simulink model "FFM_Punch"  (R2017a)
settings: Solver=ode3  StartTime=0.0  StopTime=timesteps  FixedStep=data.SIM.Ts  RelTol=1e-3  EnableMultiTasking=on
values from neighbouring files (symbols this model uses):
  data =     [dakota_config.mat]
  downshift_map = data.TCU.upshift.veh_spd_default    [Simulation_results.m]
  upshift_map = data.TCU.upshift.veh_spd_default    [Simulation_results.m]
undefined symbols (not defined in the file or in its folder): air_density, Cd, DiscIntNeverNeededParam, fr_crankshaft, fr_speed_values, g, i_FD, ICE, Low_Ratio, M_Eng_Max, M_Eng_Max_Max, M_Eng_Max_Rpm, mt2m_f, mu_Roll_C0, mu_Roll_C1, mu_Roll_C2, Mv, n_Idle_Eng, Overdrive_Ratio, Re, S_eff_drag, Ts
(part 10 of 15)

== system FFM_Punch/Driver Interface/Driver Model/Driver Pedals Determination/Brake_Pedal_Determination ==
  M_Driv : Inport
  M_eng_drvSat : Inport  Port=2
  r_Overall : Inport  Port=3
  b_neut : Inport  Port=4
  Constant : Constant  Tag=Controls_Lib  Description=constant  Value=Value  OutMin=OutMin  OutMax=OutMax  OutDataTypeStr=single  SampleTime=SampleTime  FramePeriod=FramePeriod  mask(Constant){Value=0, VectorParams1D=on, SampleTime=-1, FramePeriod=inf, OutMin=[], OutMax=[], OutDataTypeStr=single, LockScale=off}
      mask prompts: Value "Simulink:blkprm_prompts:ConstConstValue"; VectorParams1D "Simulink:blkprm_prompts:AllSrcsVector1D"; SampleTime "Simulink:blkprm_prompts:AllSrcBlksSampleTime"; FramePeriod "Simulink:blkprm_prompts:AllSrcBlksFramePeriod"; OutMin "Simulink:blkprm_prompts:OutputDesignMin"; OutMax "Simulink:blkprm_prompts:OutputDesignMax"; OutDataTypeStr "Simulink:blkprm_prompts:OUTPUT_UNIFIEDDATATYPE"; LockScale "Simulink:blkprm_prompts:LockScale"
      mask help: Output the constant specified by the 'Constant value' parameter.
      mask Help: web([fileparts(which('Lib_built')) filesep 'hlp' filesep 'lib_constant' '.html'], '-helpbrowser')
      mask TypeOptions Value: Value
      mask TypeOptions VectorParams1D: VectorParams1D
      mask TypeOptions SampleTime: SampleTime
      mask TypeOptions FramePeriod: FramePeriod
      mask TypeOptions OutMin: OutMin
      mask TypeOptions OutMax: OutMax
      mask TypeOptions OutDataTypeStr: OutDataTypeStr
      mask TypeOptions LockScale: LockScale
      mask DialogControl ParameterTabVar0 Prompt: Main
      mask Display: disp(get_param(gcb,'Value'))
  Constant2 : Constant  Value=0  OutDataTypeStr=single
  Constant3 : Constant  Value=-10000  OutDataTypeStr=single
  Gain3 : Gain  Gain=-1
  Product1 : Product  Inputs=**  RndMeth=Zero
  Saturation Dynamic : Subsystem  mask(Saturation Dynamic){OutMin=[], OutMax=[], OutDataTypeStr=single, OutputDataTypeScalingMode=single, OutDataType=sfix(16), OutScaling=2^-10, LockScale=off, RndMeth=Floor, DoSatur=off}
      mask prompts: OutMin "Simulink:masks:OutputMinimum_MP"; OutMax "Simulink:masks:OutputMaximum_MP"; OutDataTypeStr "Simulink:masks:OutputDataType_MP"; OutputDataTypeScalingMode "Simulink:masks:OutputDataTypeMode_MP"; OutDataType "Simulink:masks:OutputDataTypeegFixdt116Fixdtsingle_MP"; OutScaling "Simulink:masks:OutputScalingSlopeEg29OrSlopeBias_MP"; LockScale "Simulink:masks:LockOutputDataTypeAgainstFxpTools_MP"; RndMeth "Simulink:masks:IntegerRoundingMode_MP"; DoSatur "Simulink:masks:SaturateOnIntegerOverflow_MP"
      mask help: Simulink:masks:SaturationDynamic_MD
      mask init: same as FFM_Punch/Driver Interface/Driver Model-_old/Driver Pedal Behaviour/Saturation Dynamic
      mask Callback OutDataTypeStr: fixptdialog(gcbh)
      mask TypeOptions OutputDataTypeScalingMode: double | single | int8 | uint8 | int16 | uint16 | int32 | uint32 | Specify via dialog | Same as second input
      mask Callback OutputDataTypeScalingMode: fixptdialog(gcbh)
      mask Callback OutDataType: fixptdialog(gcbh)
      mask TypeOptions RndMeth: Simulink:masks:Ceiling | Simulink:masks:Convergent | Simulink:masks:Floor | Simulink:masks:Nearest | Simulink:masks:Round | Simulink:masks:Simplest | Simulink:masks:Zero
      mask Display: plot([0.15 0.85],[.5 .5],[.5 .5],[0.05 0.95],0.15+0.7*[0 .25 .75 1],0.05+0.9*[.25 .25 .75 .75]);
  Sum2 : Sum  Inputs=-+  OutDataTypeStr=Inherit: Inherit via back propagation
  Switch : Switch  Tag=Controls_Lib  Description=Switch  Criteria=u2 ~= 0  Threshold=Threshold  OutMin=OutMin  OutMax=OutMax  OutDataTypeStr=Inherit: Inherit via back propagation  RndMeth=Zero  ZeroCross=off  SampleTime=SampleTime  InputSameDT=on  mask(Switch){Criteria=u2 ~= 0, Threshold=0.5, ZeroCross=off, SampleTime=-1, InputSameDT=on, OutMin=[], OutMax=[], OutDataTypeStr=Inherit: Inherit via back propagation, LockScale=off, RndMeth=Zero, SaturateOnIntegerOverflow=off, AllowDiffInputSizes=off}
      mask prompts: Criteria "Criteria for passing first input:"; ZeroCross "Enable zero-crossing detection"; SampleTime "Sample time (-1 for inherited):"; InputSameDT "Require all data port inputs to have the same data type"; OutMin "Output minimum:"; OutMax "Output maximum:"; OutDataTypeStr "Output data type:"; LockScale "Lock output data type setting against changes by the fixed-point tools"; RndMeth "Integer rounding mode:"; SaturateOnIntegerOverflow "Saturate on integer overflow"; AllowDiffInputSizes "Allow different data input sizes (Results in variable-size output signal)"
      mask help:
      | Pass through input 1 when input 2 is not equal to 0. Otherwise, pass through input 3.  The inputs are numbered top to bottom (or left to right). The input 1 pass-through criteria are input 2 not equal to 0;
      | The first and third input ports are data ports, and the second input port is the control port. The control port signal should always be a boolean signal.
      mask Help: web([fileparts(which('Lib_built')) filesep 'hlp' filesep 'lib_Switch' '.html'], '-helpbrowser')
      mask TypeOptions Criteria: Criteria
      mask TypeOptions Threshold: Threshold
      mask TypeOptions ZeroCross: ZeroCross
      mask TypeOptions SampleTime: SampleTime
      mask TypeOptions InputSameDT: InputSameDT
      mask TypeOptions OutMin: OutMin
      mask TypeOptions OutMax: OutMax
      mask TypeOptions OutDataTypeStr: OutDataTypeStr
      mask TypeOptions LockScale: LockScale
      mask TypeOptions RndMeth: RndMeth
      mask TypeOptions SaturateOnIntegerOverflow: SaturateOnIntegerOverflow
      mask TypeOptions AllowDiffInputSizes: AllowDiffInputSizes
  "brake request -> brake pedal" : Lookup  InputValues=|  Table=|  LookUpMeth=Interpolation-Use End Values
      InputValues=|
      | [0
      | 
      | 
      | 200
      | 
      | 
      | 400
      | 
      | 
      | 600
      | 
      | 
      | 800
      | 
      | 
      | 1000
      | 
      | 
      | 1200
      | 
      | 
      | 1400
      | 
      | 1600
      | 
      | 
      | 1800
      | 
      | 2000]*2
      Table=|
      | [0
      | 
      | 
      | 10
      | 
      | 
      | 20
      | 
      | 
      | 30
      | 
      | 
      | 40
      | 
      | 
      | 50
      | 
      | 
      | 60
      | 
      | 
      | 70
      | 
      | 
      | 80
      | 
      | 
      | 90
      | 
      | 
      | 100]
  Driver_Brake_Request_Dcy : Outport
  wires:
  r_Overall/1 -> [r_Overall]
  M_eng_drvSat/1 -> [M_eng_drvSat]
  M_Driv/1 -> [M_Driv]
  [Driver_Brake_Request_Dcy] -> Driver_Brake_Request_Dcy/1
  Saturation Dynamic/1(y) -> Gain3/1
  Constant2/1 -> Saturation Dynamic/1(up)
  Constant3/1 -> Saturation Dynamic/3(lo)
  [M_Driv] -> Sum2/2  "wheel"
  Sum2/1 -> Saturation Dynamic/2(u)
  Gain3/1 -> "brake request -> brake pedal"/1
  "brake request -> brake pedal"/1 -> [Driver_Brake_Request_Dcy]
  [r_Overall] -> Product1/1
  [M_eng_drvSat] -> Product1/2
  Constant/1 -> Switch/3
  b_neut/1 -> Switch/2
  Switch/1 -> Sum2/1
  Product1/1 -> Switch/1

== system FFM_Punch/Driver Interface/Driver Model/Driver Pedals Determination/Preliminary_Calculations ==
  M_Driv : Inport
  n_Eng : Inport  Port=2
  r_Overall : Inport  Port=3
  v_Veh : Inport  Port=4
  Constant1 : Constant  Value=10000  OutDataTypeStr=Inherit: Inherit via back propagation
  Constant16 : Constant  Value=-100000  OutDataTypeStr=Inherit: Inherit via back propagation
  Product : Product  Inputs=*/  RndMeth=Zero
  RateLimiter : Subsystem  Tag=Controls_Lib  Description=RateLimiter  mask(Rate Limiter Dynamic){}
      mask help:
      | Limit upper and lower rates of the input signal based on the UL and LL. The rate is not limited at the first instance, output is same as the input at the first instance. 'Issat' is set to TRUE if the rate of the input signal is saturated.
      |
      | Note: The upper limit should be at least greater than or equal to the lower limit to guarantee the intended functionality.
      |
      | Inputs:
      | UL- Single [Inp/Ts]
      | Inp- Single [-]
      | LL- Single [Inp/Ts]
      |
      | outputs:
      | Out-Single [-]
      | Issat-Boolean [-]
      |
      | Where, Ts is the sample time of the model
      mask Help: web([fileparts(which('Lib_discontious')) filesep 'hlp' filesep 'lib_RateLim.html'], '-helpbrowser')
      mask Display: plot([0.15 0.95],[.5 .5],[.5 .5],[0.05 0.95],0.05+0.9*[.2 .8],0.05+0.9*[0 1]);
  Saturation1 : Saturate  UpperLimit=50  LowerLimit=data.SIM.eps
  Terminator1 : Terminator
      settings: Tag=Controls_Lib  Description=Terminator
  Terminator2 : Terminator
      settings: Tag=Controls_Lib  Description=Terminator
  Terminator3 : Terminator
      settings: Tag=Controls_Lib  Description=Terminator
  M_eng_drvSat : Outport
  wires:
  r_Overall/1 -> [r_Overall]
  n_Eng/1 -> Terminator1/1
  M_Driv/1 -> [M_Driv]
  [M_eng_drvSat] -> M_eng_drvSat/1
  Product/1 -> RateLimiter/2(Inp)  "engine"
  [M_Driv] -> Product/1
  Saturation1/1 -> Product/2
  [r_Overall] -> Saturation1/1
  Constant16/1 -> RateLimiter/3(LL)
  RateLimiter/1(Out) -> [M_eng_drvSat]
  v_Veh/1 -> Terminator2/1
  Constant1/1 -> RateLimiter/1(UL)
  RateLimiter/2(Issat) -> Terminator3/1

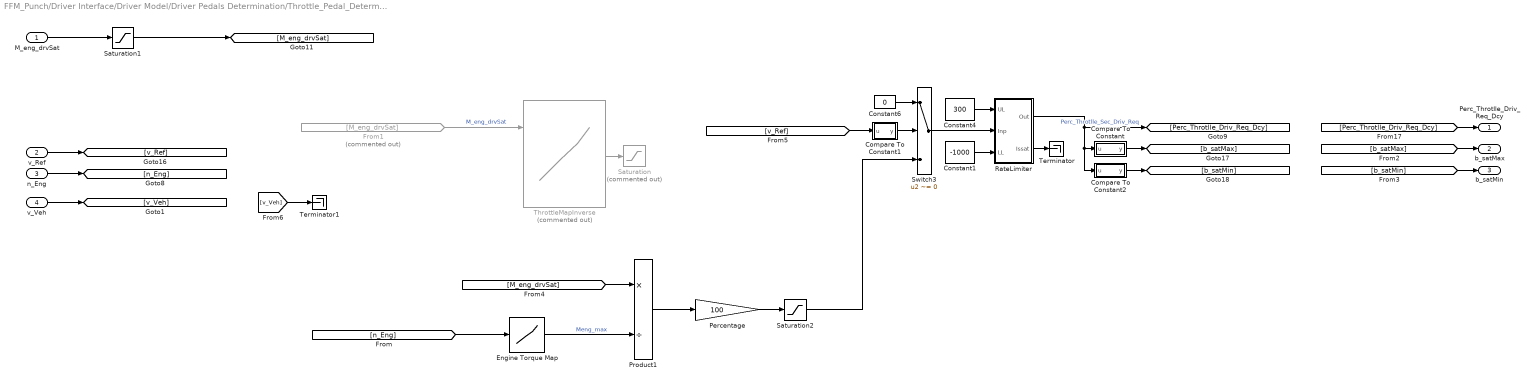
== system FFM_Punch/Driver Interface/Driver Model/Driver Pedals Determination/Throttle_Pedal_Determination ==
  M_eng_drvSat : Inport
  v_Ref : Inport  Port=2
  n_Eng : Inport  Port=3
  v_Veh : Inport  Port=4
  Compare To Constant : Subsystem  mask(Compare To Constant){relop=>=, const=100, OutDataTypeStr=boolean, ZeroCross=on}
      mask prompts: relop "Simulink:masks:Operator_MP"; const "Simulink:masks:ConstantValue_MP"; OutDataTypeStr "Simulink:masks:OutputDataType_MP"; ZeroCross "Simulink:masks:EnableZerocrossingDetection_MP"
      mask help: Simulink:masks:CompareToConstant_MD
      mask init: same as FFM_Punch/Driver Interface/Compare To Constant3
      mask TypeOptions relop: == | ~= | < | <= | >= | >
      mask TypeOptions OutDataTypeStr: Simulink:masks:uint8 | Simulink:masks:boolean
      mask Callback ZeroCross: sl('zeroCrossEnable', gcbh);
      mask Display: disp(str)
  Compare To Constant1 : Subsystem  mask(Compare To Constant){relop=<, const=1, OutDataTypeStr=boolean, ZeroCross=off}
      mask prompts: relop "Simulink:masks:Operator_MP"; const "Simulink:masks:ConstantValue_MP"; OutDataTypeStr "Simulink:masks:OutputDataType_MP"; ZeroCross "Simulink:masks:EnableZerocrossingDetection_MP"
      mask help: Simulink:masks:CompareToConstant_MD
      mask init: same as FFM_Punch/Driver Interface/Compare To Constant3
      mask TypeOptions relop: == | ~= | < | <= | >= | >
      mask TypeOptions OutDataTypeStr: Simulink:masks:uint8 | Simulink:masks:boolean
      mask Callback ZeroCross: sl('zeroCrossEnable', gcbh);
      mask Display: disp(str)
  Compare To Constant2 : Subsystem  mask(Compare To Constant){relop=<=, const=0, OutDataTypeStr=boolean, ZeroCross=on}
      mask prompts: relop "Simulink:masks:Operator_MP"; const "Simulink:masks:ConstantValue_MP"; OutDataTypeStr "Simulink:masks:OutputDataType_MP"; ZeroCross "Simulink:masks:EnableZerocrossingDetection_MP"
      mask help: Simulink:masks:CompareToConstant_MD
      mask init: same as FFM_Punch/Driver Interface/Compare To Constant3
      mask TypeOptions relop: == | ~= | < | <= | >= | >
      mask TypeOptions OutDataTypeStr: Simulink:masks:uint8 | Simulink:masks:boolean
      mask Callback ZeroCross: sl('zeroCrossEnable', gcbh);
      mask Display: disp(str)
  Constant1 : Constant  Value=-1000  OutDataTypeStr=single
  Constant4 : Constant  Value=300  OutDataTypeStr=single
  Constant6 : Constant  Value=0  OutDataTypeStr=Inherit: Inherit via back propagation
  Engine Torque Map : Lookup  InputValues=ICE.M_iceMax_XA.Value  Table=ICE.M_iceMax_M1.Value  LookUpMeth=Interpolation-Use End Values
  From1 : From  Commented=on  GotoTag=M_eng_drvSat
  Percentage : Gain  Gain=100
  Product1 : Product  Inputs=*/  SaturateOnIntegerOverflow=on  RndMeth=Zero  InputSameDT=on  OutDataTypeStr=Inherit: Same as first input
  RateLimiter : Subsystem  Tag=Controls_Lib  Description=RateLimiter  mask(Rate Limiter Dynamic){}
      mask help:
      | Limit upper and lower rates of the input signal based on the UL and LL. The rate is not limited at the first instance, output is same as the input at the first instance. 'Issat' is set to TRUE if the rate of the input signal is saturated.
      |
      | Note: The upper limit should be at least greater than or equal to the lower limit to guarantee the intended functionality.
      |
      | Inputs:
      | UL- Single [Inp/Ts]
      | Inp- Single [-]
      | LL- Single [Inp/Ts]
      |
      | outputs:
      | Out-Single [-]
      | Issat-Boolean [-]
      |
      | Where, Ts is the sample time of the model
      settings: PreCopyFcn=error('This MBD-Library block is outdated and replaced with an updated version. Please use the updated block from the MBD-Library (outdated blocks are colored in red).')
      mask Help: web([fileparts(which('Lib_discontious')) filesep 'hlp' filesep 'lib_RateLim.html'], '-helpbrowser')
      mask Display: plot([0.15 0.95],[.5 .5],[.5 .5],[0.05 0.95],0.05+0.9*[.2 .8],0.05+0.9*[0 1]);
  Saturation : Saturate  Commented=on  UpperLimit=100  LowerLimit=0
  Saturation1 : Saturate  UpperLimit=max(ICE.M_iceMax_M1.Value)  LowerLimit=0
  Saturation2 : Saturate  UpperLimit=100  LowerLimit=0
  Switch3 : Switch  Criteria=u2 ~= 0  Threshold=0.5  RndMeth=Zero  InputSameDT=on
  Terminator : Terminator
      settings: Tag=Controls_Lib  Description=Terminator
  Terminator1 : Terminator
      settings: Tag=Controls_Lib  Description=Terminator
  ThrottleMapInverse : Lookup_n-D  Commented=on  BreakpointsForDimension1=PedalMapInv_Data(1,2:end)  BreakpointsForDimension2=PedalMapInv_Data(2:end,1)  IndexSearchMethod=Linear search  BeginIndexSearchUsingPreviousIndexResult=on  Table=PedalMapInv_Data(2:end,2:end)  UseLastTableValue=on  RndMeth=Simplest  InputSameDT=on
  Perc_Throtlle_Driv_Req_Dcy : Outport
  b_satMax : Outport  Port=2
  b_satMin : Outport  Port=3
  wires:
  v_Ref/1 -> [v_Ref]
  M_eng_drvSat/1 -> Saturation1/1
  [Perc_Throtlle_Driv_Req_Dcy] -> Perc_Throtlle_Driv_Req_Dcy/1
  From1/1 -> ThrottleMapInverse/1  "M_eng_drvSat"
  ThrottleMapInverse/1 -> Saturation/1
  Compare To Constant1/1(y) -> Switch3/2
  [v_Ref] -> Compare To Constant1/1(u)
  Constant6/1 -> Switch3/1
  Switch3/1 -> RateLimiter/2(Inp)
  Constant4/1 -> RateLimiter/1(UL)
  Constant1/1 -> RateLimiter/3(LL)
  RateLimiter/1(Out) -> [Perc_Throtlle_Driv_Req_Dcy], Compare To Constant/1(u), Compare To Constant2/1(u)  "Perc_Throtlle_Sec_Driv_Req"
  Compare To Constant/1(y) -> [b_satMax]
  Compare To Constant2/1(y) -> [b_satMin]
  [b_satMax] -> b_satMax/1
  [b_satMin] -> b_satMin/1
  n_Eng/1 -> [n_Eng]
  RateLimiter/2(Issat) -> Terminator/1
  v_Veh/1 -> [v_Veh]
  Saturation1/1 -> [M_eng_drvSat]
  [n_Eng] -> Engine Torque Map/1
  Engine Torque Map/1 -> Product1/2  "Meng_max"
  Product1/1 -> Percentage/1
  [M_eng_drvSat] -> Product1/1
  Percentage/1 -> Saturation2/1
  Saturation2/1 -> Switch3/3
  [v_Veh] -> Terminator1/1

== system FFM_Punch/Driver Interface/Driver Model/Final PID Computation/Anti windup ==
  b_satMax : Inport
  b_satMin : Inport  Port=2
  v_ErrorIn : Inport  Port=3
  Constant1 : Constant  Value=0  OutDataTypeStr=Inherit: Inherit via back propagation  SampleTime=-1
  Constant81 : Constant  Value=0  OutDataTypeStr=Inherit: Inherit via back propagation  SampleTime=-1
  MinMax1 : MinMax  Function=max  Inputs=2  OutDataTypeStr=Inherit: Inherit via back propagation
  MinMax8 : MinMax  Inputs=2  OutDataTypeStr=Inherit: Inherit via back propagation
  Switch : Switch  Threshold=1  OutDataTypeStr=Inherit: Inherit via back propagation
  Switch1 : Switch  Threshold=1  OutDataTypeStr=Inherit: Inherit via back propagation
  v_ErrorOut : Outport
  wires:
  v_ErrorIn/1 -> Switch/3, MinMax8/1
  b_satMax/1 -> Switch/2
  b_satMin/1 -> Switch1/2
  MinMax1/1 -> Switch1/1
  Switch/1 -> Switch1/3, MinMax1/1
  Constant1/1 -> MinMax1/2
  MinMax8/1 -> Switch/1
  Switch1/1 -> v_ErrorOut/1
  Constant81/1 -> MinMax8/2

== system FFM_Punch/Driver Interface/Driver Model/Final PID Computation/Compare To Constant3 ==
  u : Inport
  Compare : RelationalOperator  OutDataTypeStr=boolean  ZeroCross=off  RndMeth=Nearest  InputSameDT=on
  Constant : Constant  DisableCoverage=on  Value=const  OutDataTypeStr=Inherit: Inherit via back propagation
  y : Outport
  wires:
  u/1 -> Compare/1
  Constant/1 -> Compare/2
  Compare/1 -> y/1

== system FFM_Punch/Driver Interface/Driver Model/Final Pedal Coordination/RateLimiter ==
  UL : Inport  Tag=Controls_Lib_V1.0  OutDataTypeStr=single  Interpolate=off
  Inp : Inport  Tag=Controls_Lib_V1.0  Port=2  OutDataTypeStr=single  Interpolate=off
  LL : Inport  Tag=Controls_Lib_V1.0  Port=3  OutDataTypeStr=single  Interpolate=off
  AddSub : Sum  Tag=Controls_Lib_V1.0  Inputs=+-  CollapseDim=CollapseDim  AccumDataTypeStr=single  OutMin=OutMin  OutMax=OutMax  OutDataTypeStr=single  RndMeth=Nearest  SampleTime=SampleTime  InputSameDT=on  mask(AddSub){IconShape=rectangular, Inputs=+-, CollapseMode=All dimensions, CollapseDim=1, SampleTime=-1, InputSameDT=on, AccumDataTypeStr=single, OutMin=[], OutMax=[], OutDataTypeStr=single, LockScale=off, RndMeth=Nearest, SaturateOnIntegerOverflow=off}
      mask prompts: IconShape "Icon shape:"; Inputs "List of signs:"; CollapseMode "Sum over:"; CollapseDim "Dimension:"; SampleTime "Sample time (-1 for inherited):"; InputSameDT "Require all inputs to have the same data type"; AccumDataTypeStr "Accumulator data type:"; OutMin "Output minimum:"; OutMax "Output maximum:"; OutDataTypeStr "Output data type:"; LockScale "Lock data type settings against changes by the fixed-point tools"; RndMeth "Integer rounding mode:"; SaturateOnIntegerOverflow "Saturate on integer overflow"
      mask help:
      | Add or subtract inputs.  Specify one of the following:
      | a) string containing + or - for each input port, | for spacer between ports (e.g. ++|-|++)
      | b) scalar, >= 1, specifies the number of input ports to be summed.
      | When there is only one input port, add or subtract elements over all dimensions or one specified dimension
      mask Help: web([fileparts(which('Lib_built')) filesep 'hlp' filesep 'lib_AddSub' '.html'], '-helpbrowser')
      mask TypeOptions IconShape: IconShape
      mask TypeOptions Inputs: Inputs
      mask TypeOptions CollapseMode: CollapseMode
      mask TypeOptions CollapseDim: CollapseDim
      mask TypeOptions SampleTime: SampleTime
      mask TypeOptions InputSameDT: InputSameDT
      mask TypeOptions AccumDataTypeStr: AccumDataTypeStr
      mask TypeOptions OutMin: OutMin
      mask TypeOptions OutMax: OutMax
      mask TypeOptions OutDataTypeStr: OutDataTypeStr
      mask TypeOptions LockScale: LockScale
      mask TypeOptions RndMeth: RndMeth
      mask TypeOptions SaturateOnIntegerOverflow: SaturateOnIntegerOverflow
  AddSub1 : Sum  Tag=Controls_Lib_V1.0  CollapseDim=CollapseDim  AccumDataTypeStr=single  OutMin=OutMin  OutMax=OutMax  OutDataTypeStr=single  RndMeth=Nearest  SampleTime=SampleTime  InputSameDT=on  mask(AddSub){IconShape=rectangular, Inputs=++, CollapseMode=All dimensions, CollapseDim=1, SampleTime=-1, InputSameDT=on, AccumDataTypeStr=single, OutMin=[], OutMax=[], OutDataTypeStr=single, LockScale=off, RndMeth=Nearest, SaturateOnIntegerOverflow=off}
      mask prompts: IconShape "Icon shape:"; Inputs "List of signs:"; CollapseMode "Sum over:"; CollapseDim "Dimension:"; SampleTime "Sample time (-1 for inherited):"; InputSameDT "Require all inputs to have the same data type"; AccumDataTypeStr "Accumulator data type:"; OutMin "Output minimum:"; OutMax "Output maximum:"; OutDataTypeStr "Output data type:"; LockScale "Lock data type settings against changes by the fixed-point tools"; RndMeth "Integer rounding mode:"; SaturateOnIntegerOverflow "Saturate on integer overflow"
      mask help:
      | Add or subtract inputs.  Specify one of the following:
      | a) string containing + or - for each input port, | for spacer between ports (e.g. ++|-|++)
      | b) scalar, >= 1, specifies the number of input ports to be summed.
      | When there is only one input port, add or subtract elements over all dimensions or one specified dimension
      mask Help: web([fileparts(which('Lib_built')) filesep 'hlp' filesep 'lib_AddSub' '.html'], '-helpbrowser')
      mask TypeOptions IconShape: IconShape
      mask TypeOptions Inputs: Inputs
      mask TypeOptions CollapseMode: CollapseMode
      mask TypeOptions CollapseDim: CollapseDim
      mask TypeOptions SampleTime: SampleTime
      mask TypeOptions InputSameDT: InputSameDT
      mask TypeOptions AccumDataTypeStr: AccumDataTypeStr
      mask TypeOptions OutMin: OutMin
      mask TypeOptions OutMax: OutMax
      mask TypeOptions OutDataTypeStr: OutDataTypeStr
      mask TypeOptions LockScale: LockScale
      mask TypeOptions RndMeth: RndMeth
      mask TypeOptions SaturateOnIntegerOverflow: SaturateOnIntegerOverflow
  AddSub2 : Sum  Tag=Controls_Lib_V1.0  CollapseDim=CollapseDim  AccumDataTypeStr=single  OutMin=OutMin  OutMax=OutMax  OutDataTypeStr=single  RndMeth=Nearest  SampleTime=SampleTime  InputSameDT=on  mask(AddSub){IconShape=rectangular, Inputs=++, CollapseMode=All dimensions, CollapseDim=1, SampleTime=-1, InputSameDT=on, AccumDataTypeStr=single, OutMin=[], OutMax=[], OutDataTypeStr=single, LockScale=off, RndMeth=Nearest, SaturateOnIntegerOverflow=off}
      mask prompts: IconShape "Icon shape:"; Inputs "List of signs:"; CollapseMode "Sum over:"; CollapseDim "Dimension:"; SampleTime "Sample time (-1 for inherited):"; InputSameDT "Require all inputs to have the same data type"; AccumDataTypeStr "Accumulator data type:"; OutMin "Output minimum:"; OutMax "Output maximum:"; OutDataTypeStr "Output data type:"; LockScale "Lock data type settings against changes by the fixed-point tools"; RndMeth "Integer rounding mode:"; SaturateOnIntegerOverflow "Saturate on integer overflow"
      mask help:
      | Add or subtract inputs.  Specify one of the following:
      | a) string containing + or - for each input port, | for spacer between ports (e.g. ++|-|++)
      | b) scalar, >= 1, specifies the number of input ports to be summed.
      | When there is only one input port, add or subtract elements over all dimensions or one specified dimension
      mask Help: web([fileparts(which('Lib_built')) filesep 'hlp' filesep 'lib_AddSub' '.html'], '-helpbrowser')
      mask TypeOptions IconShape: IconShape
      mask TypeOptions Inputs: Inputs
      mask TypeOptions CollapseMode: CollapseMode
      mask TypeOptions CollapseDim: CollapseDim
      mask TypeOptions SampleTime: SampleTime
      mask TypeOptions InputSameDT: InputSameDT
      mask TypeOptions AccumDataTypeStr: AccumDataTypeStr
      mask TypeOptions OutMin: OutMin
      mask TypeOptions OutMax: OutMax
      mask TypeOptions OutDataTypeStr: OutDataTypeStr
      mask TypeOptions LockScale: LockScale
      mask TypeOptions RndMeth: RndMeth
      mask TypeOptions SaturateOnIntegerOverflow: SaturateOnIntegerOverflow
  AddSub3 : Sum  Tag=Controls_Lib_V1.0  Inputs=-+  CollapseDim=CollapseDim  AccumDataTypeStr=single  OutMin=OutMin  OutMax=OutMax  OutDataTypeStr=single  RndMeth=Nearest  SampleTime=SampleTime  InputSameDT=on  mask(AddSub){IconShape=rectangular, Inputs=-+, CollapseMode=All dimensions, CollapseDim=1, SampleTime=-1, InputSameDT=on, AccumDataTypeStr=single, OutMin=[], OutMax=[], OutDataTypeStr=single, LockScale=off, RndMeth=Nearest, SaturateOnIntegerOverflow=off}
      mask prompts: IconShape "Icon shape:"; Inputs "List of signs:"; CollapseMode "Sum over:"; CollapseDim "Dimension:"; SampleTime "Sample time (-1 for inherited):"; InputSameDT "Require all inputs to have the same data type"; AccumDataTypeStr "Accumulator data type:"; OutMin "Output minimum:"; OutMax "Output maximum:"; OutDataTypeStr "Output data type:"; LockScale "Lock data type settings against changes by the fixed-point tools"; RndMeth "Integer rounding mode:"; SaturateOnIntegerOverflow "Saturate on integer overflow"
      mask help:
      | Add or subtract inputs.  Specify one of the following:
      | a) string containing + or - for each input port, | for spacer between ports (e.g. ++|-|++)
      | b) scalar, >= 1, specifies the number of input ports to be summed.
      | When there is only one input port, add or subtract elements over all dimensions or one specified dimension
      mask Help: web([fileparts(which('Lib_built')) filesep 'hlp' filesep 'lib_AddSub' '.html'], '-helpbrowser')
      mask TypeOptions IconShape: IconShape
      mask TypeOptions Inputs: Inputs
      mask TypeOptions CollapseMode: CollapseMode
      mask TypeOptions CollapseDim: CollapseDim
      mask TypeOptions SampleTime: SampleTime
      mask TypeOptions InputSameDT: InputSameDT
      mask TypeOptions AccumDataTypeStr: AccumDataTypeStr
      mask TypeOptions OutMin: OutMin
      mask TypeOptions OutMax: OutMax
      mask TypeOptions OutDataTypeStr: OutDataTypeStr
      mask TypeOptions LockScale: LockScale
      mask TypeOptions RndMeth: RndMeth
      mask TypeOptions SaturateOnIntegerOverflow: SaturateOnIntegerOverflow
  Constant : Constant  Tag=Controls_Lib_V1.0  Value=Value  VectorParams1D=off  OutMin=OutMin  OutMax=OutMax  OutDataTypeStr=Inherit: Inherit via back propagation  SampleTime=SampleTime  FramePeriod=FramePeriod  mask(Constant){Value=0.5, VectorParams1D=off, SampleTime=-1, FramePeriod=inf, OutMin=[], OutMax=[], OutDataTypeStr=Inherit: Inherit via back propagation, LockScale=off}
      mask prompts: Value "Constant value:"; VectorParams1D "Interpret vector parameters as 1-D"; SampleTime "Sample time:"; FramePeriod "Frame period:"; OutMin "Output minimum:"; OutMax "Output maximum:"; OutDataTypeStr "Output data type:"; LockScale "Lock output data type setting against changes by the fixed-point tools"
      mask help: Output the constant specified by the 'Constant value' parameter.
      mask TypeOptions Value: Value
      mask TypeOptions VectorParams1D: VectorParams1D
      mask TypeOptions SampleTime: SampleTime
      mask TypeOptions FramePeriod: FramePeriod
      mask TypeOptions OutMin: OutMin
      mask TypeOptions OutMax: OutMax
      mask TypeOptions OutDataTypeStr: OutDataTypeStr
      mask TypeOptions LockScale: LockScale
      mask Display: disp(get_param(gcb,'Value'))
  Constant1 : Constant  Tag=Controls_Lib  Description=constant  Value=Value  OutMin=OutMin  OutMax=OutMax  OutDataTypeStr=single  SampleTime=SampleTime  FramePeriod=FramePeriod  mask(Constant){Value=1, VectorParams1D=on, SampleTime=-1, FramePeriod=inf, OutMin=[], OutMax=[], OutDataTypeStr=single, LockScale=off}
      mask prompts: Value "Constant value:"; VectorParams1D "Interpret vector parameters as 1-D"; SampleTime "Sample time:"; FramePeriod "Frame period:"; OutMin "Output minimum:"; OutMax "Output maximum:"; OutDataTypeStr "Output data type:"; LockScale "Lock output data type setting against changes by the fixed-point tools"
      mask help: Output the constant specified by the 'Constant value' parameter.
      mask TypeOptions Value: Value
      mask TypeOptions VectorParams1D: VectorParams1D
      mask TypeOptions SampleTime: SampleTime
      mask TypeOptions FramePeriod: FramePeriod
      mask TypeOptions OutMin: OutMin
      mask TypeOptions OutMax: OutMax
      mask TypeOptions OutDataTypeStr: OutDataTypeStr
      mask TypeOptions LockScale: LockScale
      mask Display: disp(get_param(gcb,'Value'))
  Delay : Delay  Tag=Controls_Lib_V1.0  DelayLength=DelayLength  DelayLengthUpperLimit=DelayLengthUpperLimit  InitialConditionSource=Input port  InitialCondition=InitialCondition  SampleTime=SampleTime  mask(Delay){DelayLengthSource=Dialog, DelayLength=1, DelayLengthUpperLimit=100, InitialConditionSource=Input port, InitialCondition=0.0, ExternalReset=None, PreventDirectFeedthrough=off, DiagnosticForOutOfRangeDelayLength=None, RemoveProtectionDelayLength=off, InputProcessing=Elements as channels (sample based), UseCircularBuffer=off, SampleTime=-1, StateName=, StateMustResolveToSignalObject=off, CodeGenStateStorageClass=Auto, CodeGenStateStorageTypeQualifier=}
      mask prompts: DelayLengthSource "Delay length source:"; DelayLength "Delay length:"; DelayLengthUpperLimit "Delay upper limit:"; InitialConditionSource "Initial condition source:"; InitialCondition "Initial condition:"; ExternalReset "External reset:"; PreventDirectFeedthrough "Prevent direct feedthrough by increasing delay length to lower limit"; DiagnosticForOutOfRangeDelayLength "Diagnostic for out-of-range delay length:"; RemoveProtectionDelayLength "Remove protection against out-of-range delay length in generated code"; InputProcessing "Input processing:"; UseCircularBuffer "Use circular buffer for state"; SampleTime "Sample time (-1 for inherited):"; StateName "State name:"; StateMustResolveToSignalObject "State name must resolve to Simulink signal object"; CodeGenStateStorageClass "Code generation storage class:"; CodeGenStateStorageTypeQualifier "Code generation storage type qualifier:"
      mask help: Delay input by a fixed or variable number of samples. The initial output of the delay block is specified by the external input x0.
      settings: InputPortMap=u0,p4
      mask TypeOptions DelayLengthSource: DelayLengthSource
      mask TypeOptions DelayLength: DelayLength
      mask TypeOptions DelayLengthUpperLimit: DelayLengthUpperLimit
      mask TypeOptions InitialConditionSource: InitialConditionSource
      mask TypeOptions InitialCondition: InitialCondition
      mask TypeOptions ExternalReset: ExternalReset
      mask TypeOptions PreventDirectFeedthrough: PreventDirectFeedthrough
      mask TypeOptions DiagnosticForOutOfRangeDelayLength: DiagnosticForOutOfRangeDelayLength
      mask TypeOptions RemoveProtectionDelayLength: RemoveProtectionDelayLength
      mask TypeOptions InputProcessing: InputProcessing
      mask TypeOptions UseCircularBuffer: UseCircularBuffer
      mask TypeOptions SampleTime: SampleTime
      mask TypeOptions StateName: StateName
      mask TypeOptions StateMustResolveToSignalObject: StateMustResolveToSignalObject
      mask TypeOptions CodeGenStateStorageClass: CodeGenStateStorageClass
      mask TypeOptions CodeGenStateStorageTypeQualifier: CodeGenStateStorageTypeQualifier
  MulDiv : Product  Tag=Controls_Lib_V1.0  Inputs=*/  CollapseDim=CollapseDim  OutMin=OutMin  OutMax=OutMax  OutDataTypeStr=single  SampleTime=SampleTime  InputSameDT=on  mask(MulDiv){Inputs=*/, Multiplication=Element-wise(.*), CollapseMode=All dimensions, CollapseDim=1, SampleTime=-1, InputSameDT=on, OutMin=[], OutMax=[], OutDataTypeStr=single, LockScale=off, RndMeth=Floor, SaturateOnIntegerOverflow=off}
      mask prompts: Inputs "Number of inputs:"; CollapseMode "Multiply over:"; CollapseDim "Dimension:"; SampleTime "Sample time (-1 for inherited):"; InputSameDT "Require all inputs to have the same data type"; OutMin "Output minimum:"; OutMax "Output maximum:"; OutDataTypeStr "Output data type:"; LockScale "Lock output data type setting against changes by the fixed-point tools"; RndMeth "Integer rounding mode:"; SaturateOnIntegerOverflow "Saturate on integer overflow"
      mask help:
      | Multiply or divide inputs element-wise. Specify one of the following:
      |  a) * or / for each input port. For example, **/* performs the operation 'u1*u2/u3*u4'.
      |  b) scalar specifies the number of input ports to be multiplied.
      | If there is only one input port and the Multiplication parameter is set to Element-wise(.*), a single * or / collapses the input signal using the specified operation.
      mask Help: web([fileparts(which('Lib_built')) filesep 'hlp' filesep 'lib_MulDiv' '.html'], '-helpbrowser')
      mask TypeOptions Inputs: Inputs
      mask TypeOptions Multiplication: Multiplication
      mask TypeOptions CollapseMode: CollapseMode
      mask TypeOptions CollapseDim: CollapseDim
      mask TypeOptions SampleTime: SampleTime
      mask TypeOptions InputSameDT: InputSameDT
      mask TypeOptions OutMin: OutMin
      mask TypeOptions OutMax: OutMax
      mask TypeOptions OutDataTypeStr: OutDataTypeStr
      mask TypeOptions LockScale: LockScale
      mask TypeOptions RndMeth: RndMeth
      mask TypeOptions SaturateOnIntegerOverflow: SaturateOnIntegerOverflow
  MulDiv1 : Product  Tag=Controls_Lib_V1.0  Inputs=**  CollapseDim=CollapseDim  OutMin=OutMin  OutMax=OutMax  OutDataTypeStr=single  SampleTime=SampleTime  InputSameDT=on  mask(MulDiv){Inputs=**, Multiplication=Element-wise(.*), CollapseMode=All dimensions, CollapseDim=1, SampleTime=-1, InputSameDT=on, OutMin=[], OutMax=[], OutDataTypeStr=single, LockScale=off, RndMeth=Floor, SaturateOnIntegerOverflow=off}
      mask prompts: Inputs "Number of inputs:"; CollapseMode "Multiply over:"; CollapseDim "Dimension:"; SampleTime "Sample time (-1 for inherited):"; InputSameDT "Require all inputs to have the same data type"; OutMin "Output minimum:"; OutMax "Output maximum:"; OutDataTypeStr "Output data type:"; LockScale "Lock output data type setting against changes by the fixed-point tools"; RndMeth "Integer rounding mode:"; SaturateOnIntegerOverflow "Saturate on integer overflow"
      mask help:
      | Multiply or divide inputs element-wise. Specify one of the following:
      |  a) * or / for each input port. For example, **/* performs the operation 'u1*u2/u3*u4'.
      |  b) scalar specifies the number of input ports to be multiplied.
      | If there is only one input port and the Multiplication parameter is set to Element-wise(.*), a single * or / collapses the input signal using the specified operation.
      mask Help: web([fileparts(which('Lib_built')) filesep 'hlp' filesep 'lib_MulDiv' '.html'], '-helpbrowser')
      mask TypeOptions Inputs: Inputs
      mask TypeOptions Multiplication: Multiplication
      mask TypeOptions CollapseMode: CollapseMode
      mask TypeOptions CollapseDim: CollapseDim
      mask TypeOptions SampleTime: SampleTime
      mask TypeOptions InputSameDT: InputSameDT
      mask TypeOptions OutMin: OutMin
      mask TypeOptions OutMax: OutMax
      mask TypeOptions OutDataTypeStr: OutDataTypeStr
      mask TypeOptions LockScale: LockScale
      mask TypeOptions RndMeth: RndMeth
      mask TypeOptions SaturateOnIntegerOverflow: SaturateOnIntegerOverflow
  MulDiv2 : Product  Tag=Controls_Lib_V1.0  Inputs=***  CollapseDim=CollapseDim  OutMin=OutMin  OutMax=OutMax  OutDataTypeStr=single  SampleTime=SampleTime  InputSameDT=on  mask(MulDiv){Inputs=***, Multiplication=Element-wise(.*), CollapseMode=All dimensions, CollapseDim=1, SampleTime=-1, InputSameDT=on, OutMin=[], OutMax=[], OutDataTypeStr=single, LockScale=off, RndMeth=Floor, SaturateOnIntegerOverflow=off}
      mask prompts: Inputs "Number of inputs:"; CollapseMode "Multiply over:"; CollapseDim "Dimension:"; SampleTime "Sample time (-1 for inherited):"; InputSameDT "Require all inputs to have the same data type"; OutMin "Output minimum:"; OutMax "Output maximum:"; OutDataTypeStr "Output data type:"; LockScale "Lock output data type setting against changes by the fixed-point tools"; RndMeth "Integer rounding mode:"; SaturateOnIntegerOverflow "Saturate on integer overflow"
      mask help:
      | Multiply or divide inputs element-wise. Specify one of the following:
      |  a) * or / for each input port. For example, **/* performs the operation 'u1*u2/u3*u4'.
      |  b) scalar specifies the number of input ports to be multiplied.
      | If there is only one input port and the Multiplication parameter is set to Element-wise(.*), a single * or / collapses the input signal using the specified operation.
      mask Help: web([fileparts(which('Lib_built')) filesep 'hlp' filesep 'lib_MulDiv' '.html'], '-helpbrowser')
      mask TypeOptions Inputs: Inputs
      mask TypeOptions Multiplication: Multiplication
      mask TypeOptions CollapseMode: CollapseMode
      mask TypeOptions CollapseDim: CollapseDim
      mask TypeOptions SampleTime: SampleTime
      mask TypeOptions InputSameDT: InputSameDT
      mask TypeOptions OutMin: OutMin
      mask TypeOptions OutMax: OutMax
      mask TypeOptions OutDataTypeStr: OutDataTypeStr
      mask TypeOptions LockScale: LockScale
      mask TypeOptions RndMeth: RndMeth
      mask TypeOptions SaturateOnIntegerOverflow: SaturateOnIntegerOverflow
  MulDiv3 : Product  Tag=Controls_Lib_V1.0  Inputs=*/  CollapseDim=CollapseDim  OutMin=OutMin  OutMax=OutMax  OutDataTypeStr=single  SampleTime=SampleTime  InputSameDT=on  mask(MulDiv){Inputs=*/, Multiplication=Element-wise(.*), CollapseMode=All dimensions, CollapseDim=1, SampleTime=-1, InputSameDT=on, OutMin=[], OutMax=[], OutDataTypeStr=single, LockScale=off, RndMeth=Floor, SaturateOnIntegerOverflow=off}
      mask prompts: Inputs "Number of inputs:"; CollapseMode "Multiply over:"; CollapseDim "Dimension:"; SampleTime "Sample time (-1 for inherited):"; InputSameDT "Require all inputs to have the same data type"; OutMin "Output minimum:"; OutMax "Output maximum:"; OutDataTypeStr "Output data type:"; LockScale "Lock output data type setting against changes by the fixed-point tools"; RndMeth "Integer rounding mode:"; SaturateOnIntegerOverflow "Saturate on integer overflow"
      mask help:
      | Multiply or divide inputs element-wise. Specify one of the following:
      |  a) * or / for each input port. For example, **/* performs the operation 'u1*u2/u3*u4'.
      |  b) scalar specifies the number of input ports to be multiplied.
      | If there is only one input port and the Multiplication parameter is set to Element-wise(.*), a single * or / collapses the input signal using the specified operation.
      mask Help: web([fileparts(which('Lib_built')) filesep 'hlp' filesep 'lib_MulDiv' '.html'], '-helpbrowser')
      mask TypeOptions Inputs: Inputs
      mask TypeOptions Multiplication: Multiplication
      mask TypeOptions CollapseMode: CollapseMode
      mask TypeOptions CollapseDim: CollapseDim
      mask TypeOptions SampleTime: SampleTime
      mask TypeOptions InputSameDT: InputSameDT
      mask TypeOptions OutMin: OutMin
      mask TypeOptions OutMax: OutMax
      mask TypeOptions OutDataTypeStr: OutDataTypeStr
      mask TypeOptions LockScale: LockScale
      mask TypeOptions RndMeth: RndMeth
      mask TypeOptions SaturateOnIntegerOverflow: SaturateOnIntegerOverflow
  SatChck : Subsystem  mask(SATURATION){}
      mask help:
      | The Saturation with Check block imposes upper and lower limits on an input signal. If the input signal is outside of these limits, saturation flag shall be raised.
      |
      | The upper limit (Max) shall be  greater than the lower limit (Min) for the saturation block to work as intended.
      mask Help: web([fileparts(which('Lib_discontious')) filesep 'hlp' filesep 'lib_SatChck.html'], '-helpbrowser')
      mask Display: plot([0 1 2 3 4 5],[0 0 0 1 1 1],[0 5],[0.5 0.5],[2.5 2.5],[0 1])
  TsInverse : SampleTimeMath  TsampMathOp=1/Ts Only  weightValue=weightValue  OutDataTypeStr=Inherit: Inherit via back propagation  mask(Sample time block){TsampMathOp=1/Ts Only, weightValue=1, TsampMathImp=Online Calculations, OutDataTypeStr=Inherit: Inherit via back propagation, RndMeth=Floor, SaturateOnIntegerOverflow=off}
      mask prompts: TsampMathOp "Operation:"; weightValue "Weight value:"; TsampMathImp "Implement using:"; OutDataTypeStr "Output data type:"; RndMeth "Integer rounding mode:"; SaturateOnIntegerOverflow "Saturate on integer overflow"
      mask help: 1 divided by the Sample time of the input signal
      mask Help: web([fileparts(which('Lib_built')) filesep 'hlp' filesep 'lib_TsInv' '.html'], '-helpbrowser')
      mask TypeOptions TsampMathOp: TsampMathOp
      mask TypeOptions weightValue: weightValue
      mask TypeOptions TsampMathImp: TsampMathImp
      mask TypeOptions OutDataTypeStr: OutDataTypeStr
      mask TypeOptions RndMeth: RndMeth
      mask TypeOptions SaturateOnIntegerOverflow: SaturateOnIntegerOverflow
  Out : Outport  Tag=Controls_Lib_V1.0  OutDataTypeStr=single  InitialOutput=0
  Issat : Outport  Tag=Controls_Lib_V1.0  Port=2  OutDataTypeStr=boolean  InitialOutput=0
  wires:
  MulDiv3/1 -> [Ts]
  TsInverse/1 -> MulDiv3/2
  Constant1/1 -> MulDiv3/1
  [Init] -> Delay/2
  Delay/1 -> [OutPrev]
  AddSub3/1 -> [Init]
  MulDiv2/1 -> AddSub3/1
  [Inp] -> AddSub3/2
  Constant/1 -> MulDiv2/3
  AddSub2/1 -> MulDiv2/2
  [LL] -> AddSub2/2
  [UL] -> AddSub2/1
  AddSub1/1 -> Delay/1, Out/1
  [Ts] -> MulDiv1/1
  [OutPrev] -> AddSub1/2
  MulDiv1/1 -> AddSub1/1
  SatChck/1(ValSat) -> MulDiv1/2
  MulDiv/1 -> SatChck/2(Inp)
  [Ts] -> MulDiv2/1, MulDiv/2
  AddSub/1 -> MulDiv/1
  SatChck/2(IsSat) -> Issat/1
  [LL] -> SatChck/3(Min)
  [UL] -> SatChck/1(Max)
  [OutPrev] -> AddSub/2
  [Inp] -> AddSub/1
  LL/1 -> [LL]
  Inp/1 -> TsInverse/1, [Inp]
  UL/1 -> [UL]

== system FFM_Punch/Driver Interface/Driver Model-_old/Driver Pedal Behaviour/Saturation Dynamic ==
  up : Inport
  u : Inport  Port=2
  lo : Inport  Port=3
  Data Type Duplicate : DataTypeDuplicate  DisableCoverage=on
  Data Type Propagation : S-Function  FunctionName=sfix_dtprop  Parameters=14,PropDataTypeMode,(getdatatypespecs(PropDataType,PropScaling,DblOver,0, 0, PropDataTypeMode, PropScalingMode)),IfRefDouble,IfRefSingle,IsSigned,NumBitsBase,NumBitsMult,NumBitsAdd,(sort(reshape(round(NumBitsAllowFinal), prod(size(NumBitsAllowFinal)),1))),PropScalingMode,ValuesUsedBestPrec,SlopeBase,SlopeMult,SlopeAdd,BiasBase,BiasMult,BiasAdd,DblOver  SFunctionDeploymentMode=off  EnableBusSupport=off  mask(Data Type Propagation){PropDataTypeMode=Inherit via propagation rule, PropDataType=fixdt(1, 16), IfRefDouble=double, IfRefSingle=single, IsSigned=IsSigned1, NumBitsBase=NumBits1, NumBitsMult=1, NumBitsAdd=0, NumBitsAllowFinal=1:128, PropScalingMode=Inherit via propagation rule, PropScaling=2^-10, ValuesUsedBestPrec=[5 -7], SlopeBase=Slope1, SlopeMult=1, SlopeAdd=0, BiasBase=Bias1, BiasMult=1, BiasAdd=0}
      mask prompts: PropDataTypeMode "Simulink:masks:x1PropagatedDataType_MP"; PropDataType "Simulink:masks:x11PropagatedDataTypeegFixdt116Fixdtsingle_MP"; IfRefDouble "Simulink:masks:x11IfAnyReferenceInputIsDoubleOutputIs_MP"; IfRefSingle "Simulink:masks:x12IfAnyReferenceInputIsSingleOutputIs_MP"; IsSigned "Simulink:masks:x13IsSigned_MP"; NumBitsBase "Simulink:masks:x141NumberofBitsBase_MP"; NumBitsMult "Simulink:masks:x142NumberofBitsMultiplicativeAdjustment_MP"; NumBitsAdd "Simulink:masks:x143NumberofBitsAdditiveAdjustment_MP"; NumBitsAllowFinal "Simulink:masks:x144NumberofBitsAllowableFinalValues_MP"; PropScalingMode "Simulink:masks:x2PropagatedScaling_MP"; PropScaling "Simulink:masks:x21PropagatedScalingSlopeEg29OrSlopeBiasEg1253_MP"; ValuesUsedBestPrec "Simulink:masks:x21ValuesUsedToDetermineBestPrecisionScaling_MP"; SlopeBase "Simulink:masks:x211SlopeBase_MP"; SlopeMult "Simulink:masks:x212SlopeMultiplicativeAdjustment_MP"; SlopeAdd "Simulink:masks:x213SlopeAdditiveAdjustment_MP"; BiasBase "Simulink:masks:x221BiasBase_MP"; BiasMult "Simulink:masks:x222BiasMultiplicativeAdjustment_MP"; BiasAdd "Simulink:masks:x223BiasAdditiveAdjustment_MP"
      mask help: Simulink:masks:DataTypePropagation_MD
      mask init:
      | DblOver = 0;
      mask TypeOptions PropDataTypeMode: Simulink:masks:SpecifyViaDialog | Simulink:masks:InheritViaPropagationRule
      mask Callback PropDataTypeMode: fixptdialog(gcbh)
      mask Callback PropDataType: fixptdialog(gcbh)
      mask TypeOptions IfRefDouble: Simulink:masks:double | Simulink:masks:single
      mask TypeOptions IfRefSingle: Simulink:masks:double | Simulink:masks:single
      mask TypeOptions IsSigned: Simulink:masks:IsSigned1 | Simulink:masks:IsSigned2 | Simulink:masks:IsSigned1OrIsSigned2 | Simulink:masks:TRUE | Simulink:masks:FALSE
      mask TypeOptions NumBitsBase: NumBits1 | NumBits2 | max([NumBits1 NumBits2]) | min([NumBits1 NumBits2]) | NumBits1+NumBits2
      mask TypeOptions PropScalingMode: Simulink:masks:SpecifyViaDialog | Simulink:masks:InheritViaPropagationRule | Simulink:masks:ObtainViaBestPrecision
      mask Callback PropScalingMode: fixptdialog(gcbh)
      mask TypeOptions SlopeBase: Slope1 | Slope2 | max([Slope1 Slope2]) | min([Slope1 Slope2]) | Slope1*Slope2 | Slope1/Slope2 | PosRange1 | PosRange2 | max([PosRange1 PosRange2]) | min([PosRange1 PosRange2]) | PosRange1*PosRange2 | PosRange1/PosRange2
      mask TypeOptions BiasBase: Bias1 | Bias2 | max([Bias1 Bias2]) | min([Bias1 Bias2]) | Bias1*Bias2 | Bias1/Bias2 | Bias1+Bias2 | Bias1-Bias2
      mask Display:
      | port_label('Input',1,'Ref1');
      | port_label('Input',2,'Ref2');
      | port_label('Input',3,'Prop');
  LowerRelop1 : RelationalOperator  DisableCoverage=on  Operator=>  OutDataTypeStr=boolean  RndMeth=Nearest
  Switch : Switch  Criteria=u2 ~= 0  OutDataTypeStr=Inherit: Inherit via back propagation  ZeroCross=off
  Switch2 : Switch  Criteria=u2 ~= 0  OutMin=OutMin  OutMax=OutMax  OutDataTypeStr=Inherit: Inherit via back propagation  ZeroCross=off
  UpperRelop : RelationalOperator  DisableCoverage=on  Operator=<  OutDataTypeStr=boolean  RndMeth=Nearest
  y : Outport  OutMin=OutMin  OutMax=OutMax
  wires:
  up/1 -> Switch2/1, LowerRelop1/2
  u/1 -> Data Type Propagation/2, Data Type Propagation/1, LowerRelop1/1, Switch/3, UpperRelop/1
  lo/1 -> Switch/1, UpperRelop/2
  Switch/1 -> Data Type Duplicate/2, Switch2/3, Data Type Propagation/3
  Switch2/1 -> Data Type Duplicate/1, y/1
  LowerRelop1/1 -> Switch2/2
  UpperRelop/1 -> Switch/2
